simulink library "discrete_time_low_pass_filter"  (R2025b)
settings: Solver=VariableStepAuto  StartTime=0.0  StopTime=10.0  RelTol=1e-3
undefined symbols (not defined in the file): ts
settings Model: Creator=dbagn  LastModifiedBy=dbagn

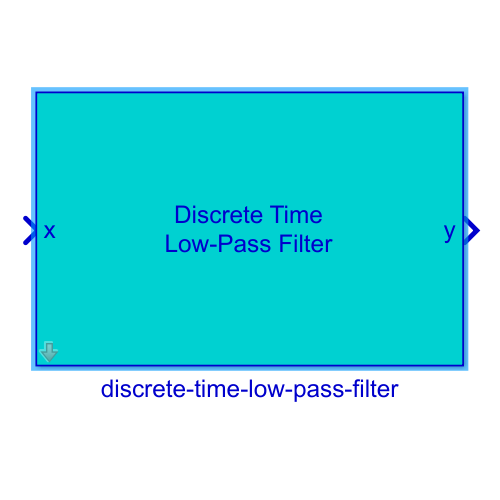
[thumbnail: Simulink's stored preview of the top-level diagram]
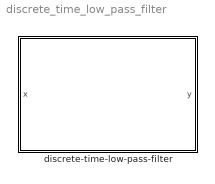
== system discrete_time_low_pass_filter ==
  discrete-time-low-pass-filter : Subsystem  mask{tau=1e-3, ts=ts}
      mask prompts: tau "time constant (s)"; ts "Sampling Time (s)"
      mask Display:
      | X = sprintf('Discrete Time\nLow-Pass Filter');
      | disp(X);
      | port_label('input', 1, 'x');
      | port_label('output', 1, 'y');

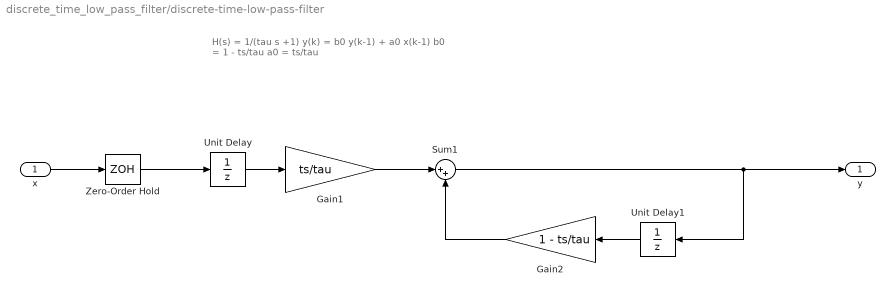
== system discrete_time_low_pass_filter/discrete-time-low-pass-filter ==
  note: H(s) = 1/(tau s +1)
      | y(k) = b0 y(k-1) + a0 x(k-1)
      | b0 = 1 - ts/tau
      | a0 = ts/tau
  x : Inport
  Gain1 : Gain  Gain=ts/tau
  Gain2 : Gain  Gain=1 - ts/tau
  Sum1 : Sum  Inputs=|++
  Unit Delay : UnitDelay  SampleTime=-1  HasFrameUpgradeWarning=on
  Unit Delay1 : UnitDelay  SampleTime=-1  HasFrameUpgradeWarning=on
  Zero-Order Hold : ZeroOrderHold  SampleTime=-1
  y : Outport
  wires:
  x/1 -> Zero-Order Hold/1
  Sum1/1 -> y/1, Unit Delay1/1
  Unit Delay/1 -> Gain1/1
  Unit Delay1/1 -> Gain2/1
  Gain2/1 -> Sum1/2
  Gain1/1 -> Sum1/1
  Zero-Order Hold/1 -> Unit Delay/1
